simulink model "Practica1"  (R2025a)
settings: Solver=VariableStepAuto  StartTime=0.0  StopTime=10.0  RelTol=1e-3

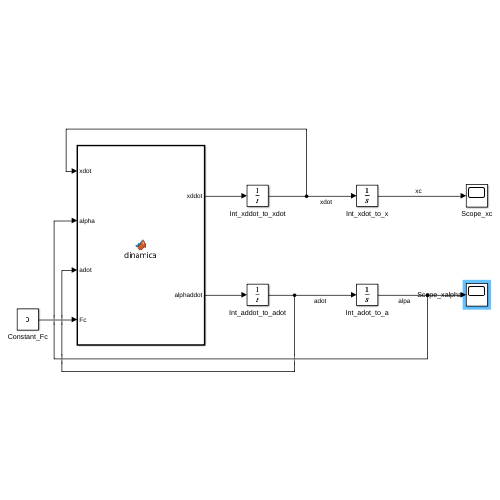
[thumbnail: Simulink's stored preview of the top-level diagram]
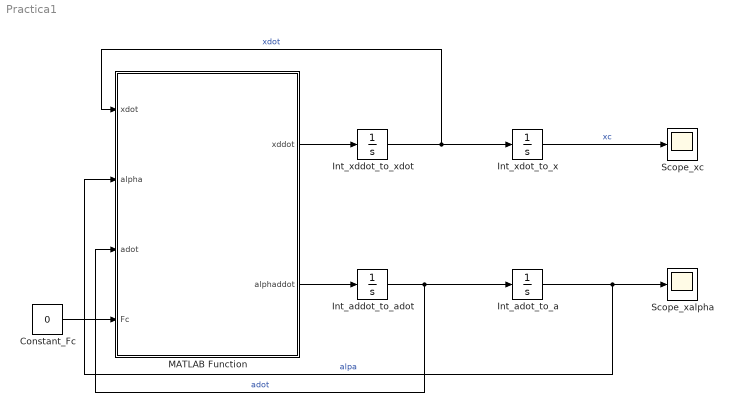
== system Practica1 ==
  Constant_Fc : Constant  Value=0
  Int_addot_to_adot : Integrator
  Int_adot_to_a : Integrator  InitialCondition=pi/180  AbsoluteTolerance=1
  Int_xddot_to_xdot : Integrator
  Int_xdot_to_x : Integrator
  MATLAB Function : MATLAB Function  TreatAsAtomicUnit=on
  Scope_xalpha : Scope
      settings: ActiveDisplayYMinimum=-58.341571609327119  ActiveDisplayYMaximum=156.56967811721978
  Scope_xc : Scope
      settings: ActiveDisplayYMinimum=-27.063388675282152  ActiveDisplayYMaximum=31.369627710280007
  wires:
  Int_xddot_to_xdot/1 -> MATLAB Function/1(xdot), Int_xdot_to_x/1  "xdot"
  Int_xdot_to_x/1 -> Scope_xc/1  "xc"
  Int_addot_to_adot/1 -> Int_adot_to_a/1, MATLAB Function/3(adot)  "adot"
  Int_adot_to_a/1 -> MATLAB Function/2(alpha), Scope_xalpha/1  "alpa"
  Constant_Fc/1 -> MATLAB Function/4(Fc)
  MATLAB Function/1(xddot) -> Int_xddot_to_xdot/1
  MATLAB Function/2(alphaddot) -> Int_addot_to_adot/1

== matlab function Practica1/MATLAB Function ==
  data: xdot input; alpha input; adot input; Fc input; xddot output; alphaddot output
function [xddot, alphaddot] = dinamica(xdot, alpha, adot, Fc)
% Dinámica del péndulo invertido en carrito
% Entradas: 
%   xdot   = velocidad del carro
%   alpha  = ángulo del péndulo (rad)
%   adot   = velocidad angular del péndulo
%   Fc     = fuerza en el carro
% Salidas:
%   xddot      = aceleración del carro
%   alphaddot  = aceleración angular del péndulo

% Parámetros del sistema (del PDF)
Ip  = 0.0079;     % kg*m^2
Mc  = 0.7031;     % kg
lp  = 0.3302;     % m
Mp  = 0.23;       % kg
Beq = 4.3;        % N*s/m
g   = 9.81;       % m/s^2
Bp  = 0.0024;     % N*m*s/rad

% Denominador común
D = (Mc+Mp)*Ip + Mc*Mp*lp^2 + (Mp^2*lp^2)*(sin(alpha)^2);

% Numerador de xddot
Nx = (Ip + Mp*lp^2)*Fc ...
     + (Mp^2*lp^2*g)*cos(alpha)*sin(alpha) ...
     - (Ip + Mp*lp^2)*Beq*xdot ...
     - (Ip*Mp*lp - Mp^2*lp^3)*(adot^2)*sin(alpha) ...
     - (Mp*lp*Bp)*adot*cos(alpha);

% Numerador de alphaddot
Na = ((Mc+Mp)*Mp*g*lp)*sin(alpha) ...
     - ((Mc+Mp)*Bp)*adot ...
     + (Fc*Mp*lp)*cos(alpha) ...
     - (Mp^2*lp^2)*(adot^2)*sin(alpha)*cos(alpha) ...
     - (Beq*Mp*lp)*xdot*cos(alpha);

% Aceleraciones
xddot = Nx / D;
alphaddot = Na / D;
end
